simulink model "Over_current_relay"  (R2024a)
settings: Solver=VariableStepAuto  StartTime=0.0  StopTime=10  RelTol=1e-3
libraries: spsACVoltageSourceLib x3, spsGroundLib x3, spsThreePhaseBreakerLib x3, spsVariableRatioTransformerLib x3, spsAsynchronousMachineSIUnitsLib x1, spsCurrentMeasurementLib x1, simulink_extras x1, spsVoltageMeasurementLib x1, sps_lib x1
settings Model: Creator=gshma  LastModifiedBy=gshma

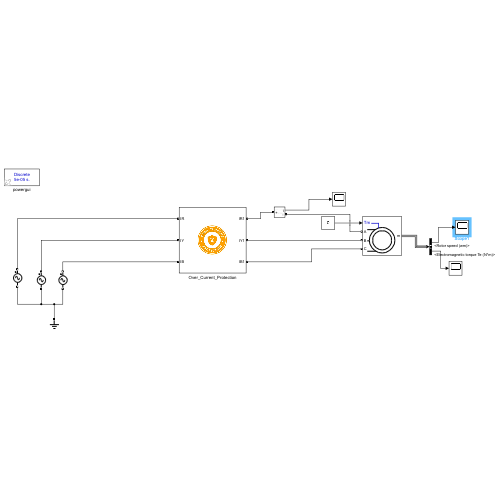
[thumbnail: Simulink's stored preview of the top-level diagram]
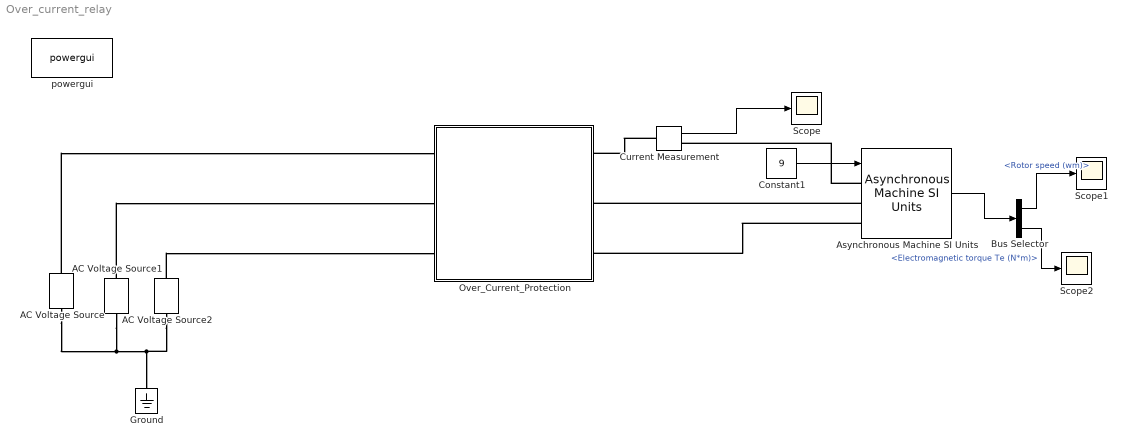
== system Over_current_relay ==
  AC Voltage Source : spsACVoltageSourceLib/AC Voltage Source  Amplitude=400  Phase=0  Frequency=50  SampleTime=0  Measurements=None  BusType=swing  Pref=10e3  Qref=0  Qmin=-inf  Qmax=+inf
  AC Voltage Source1 : spsACVoltageSourceLib/AC Voltage Source  Amplitude=400  Phase=120  Frequency=50  SampleTime=0  Measurements=None  BusType=swing  Pref=10e3  Qref=0  Qmin=-inf  Qmax=+inf
  AC Voltage Source2 : spsACVoltageSourceLib/AC Voltage Source  Amplitude=400  Phase=240  Frequency=50  SampleTime=0  Measurements=None  BusType=swing  Pref=10e3  Qref=0  Qmin=-inf  Qmax=+inf
  Asynchronous Machine SI Units : spsAsynchronousMachineSIUnitsLib/Asynchronous Machine SI Units  RotorType=Squirrel-cage  PresetModel="15:  5.4 HP (4KW)   400 V  50Hz 1430 RPM"  MechanicalLoad=Torque Tm  ShowDetailedParameters=on  ReferenceFrame=Rotor  Units=SI  MeasurementBus=off  NominalParameters=[4000 400 50]  VoltageRatio=1  Stator=[1.405 0.005839]  Rotor=[1.395 0.005839]  Cage1=[0.4155 0.002066]  Cage2=[0.4168 0.0003495]  Lm=0.1722  Mechanical=[0.0131 0.002985 2]  PolePairs=2  InitialConditions=[0 0 0 0 0 0 0 0]  SimulateSaturation=off  Saturation=[14.03593122, 27.81365428, 53.79336849, 72.68890987, 97.98006896, 148.6815601, 215.7428561, 302.9841135, 428.7778367 ; 230, 322, 414, 460, 506, 552, 598, 644, 690]  LoadFlowParameters=1492000  TsPowergui=0  TsBlock=-1  IterativeModel=Trapezoidal non iterative  IterativeDiscreteModel=Trapezoidal non iterative  Pmec=1.492e+006
  Bus Selector : BusSelector  OutputSignals=Mechanical.Rotor speed (wm),Mechanical.Electromagnetic torque Te (N*m)
  Constant1 : Constant  Value=9  SampleTime=0.001
  Current Measurement : spsCurrentMeasurementLib/Current Measurement  PhasorSimulation=off  OutputType=Complex  PSBequivalent=0
  Ground : spsGroundLib/Ground  LConnTagsString=a
  Over_Current_Protection : Subsystem
      mask Display: image('ovv.png', [0,0,0,0,50,50]);
  Scope : Scope
  Scope1 : Scope
  Scope2 : Scope
  powergui : sps_lib/powergui  Priority=1  SimulationMode=Discrete  SampleTime=50e-6  frequency=60  Iterations=50  frequencyindice=50  Pbase=100e6  ErrMax=1e-4  UnitsV=kV  UnitsW=MW  buscounter=0  FunctionMessages=off  echomessages=off  EnableUseOfTLC=off  CurrentSourceSwitches=off  DisableSnubberDevices=off  DisableRonSwitches=off  DisableVfSwitches=off  DisplayEquations=off  AutomaticDiscreteSolvers=off  SolverType=Tustin/Backward Euler (TBE)  Interpol=off  ExternalGateDelay=off  methode=off  Ts=100  x0status=blocks  SPID=on  SwTol=0  HookPort=off  NonlinearTolerance=1e-4  nMaxIteration=100  ContinueOnMaxIteration=off  RestoreLinks=warning  ResistiveCurrentMeasurement=off  Frange=[0:2:500]  Ylog=off  Xlog=on  ShowGrid=off  save=off  variable=ZData  structure=0  ZoomFFT=off  StartTime=0.0  cycles=1  DisplayStyle=1  fundamental=60  FreqAxis=off  MaxFrequency=1000  frequencyindicesteady=1  RmsSteady=1  display=off
  wires:
  Current Measurement/1 -> Scope/1
  Constant1/1 -> Asynchronous Machine SI Units/1
  Asynchronous Machine SI Units/1 -> Bus Selector/1
  Bus Selector/1 -> Scope1/1  "<Rotor speed (wm)>"
  Bus Selector/2 -> Scope2/1  "<Electromagnetic torque Te (N*m)>"
  connections:
  AC Voltage Source/RConn1 -- Over_Current_Protection/LConn1
  AC Voltage Source1/RConn1 -- Over_Current_Protection/LConn2
  AC Voltage Source2/RConn1 -- Over_Current_Protection/LConn3
  Current Measurement/LConn1 -- Over_Current_Protection/RConn1
  Asynchronous Machine SI Units/LConn1 -- Current Measurement/RConn1
  Asynchronous Machine SI Units/LConn2 -- Over_Current_Protection/RConn2
  Asynchronous Machine SI Units/LConn3 -- Over_Current_Protection/RConn3
  AC Voltage Source/LConn1 -- AC Voltage Source1/LConn1 -- AC Voltage Source2/LConn1 -- Ground/LConn1

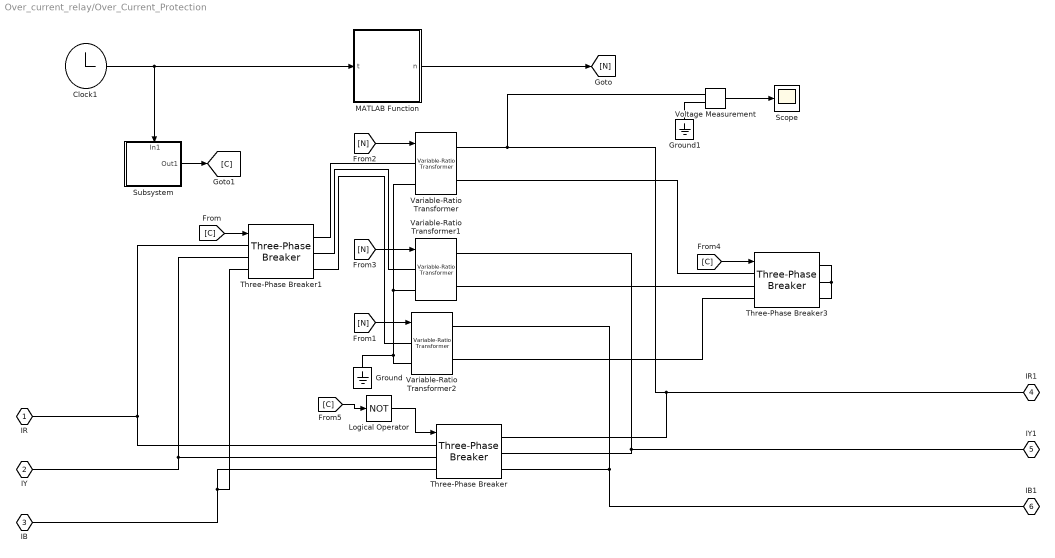
== system Over_current_relay/Over_Current_Protection ==
  Clock1 : Clock
      settings: Decimation=1000
  Ground : spsGroundLib/Ground  LConnTagsString=a
  Ground1 : spsGroundLib/Ground  LConnTagsString=a
  Logical Operator : Logic  Operator=NOT  AllPortsSameDT=off  OutDataTypeStr=boolean
  MATLAB Function : MATLAB Function  TreatAsAtomicUnit=on
  Scope : Scope
  Subsystem : Subsystem
      settings: PortSchema="{\"entries\":[{\"content\":{\"sides\":[{\"content\":{},\"type\":\"ConnectorPlacement.EquallySpacedRectSide\",\"uuid\":\"eeea18b9-380b-488c-afba-283aabc25f85\"},{\"content\":{\"connectorIds\":[\"Out1\"],\"side\":\"RIGHT\"},\"type\":\"ConnectorPlacement.EquallySpacedRectSide\",\"uuid\":\"b5cdad00-14f9-426f-8cac-c80f210bc817\"},{\"content\":{\"connectorIds\":[\"In1\"],\"side\":\"TOP\"},\"type\":\"ConnectorPlacement.EquallySpacedRectSide\",\"uuid\":\"d8660c5f-ab56-4d32-b432-a9ce1bc682f2\"}]},\"type\":\"ConnectorPlacement.EquallySpacedConnector\",\"uuid\":\"80a26fe6-a8a6-4d75-a5f0-c797e7c8950d\"}],\"packageUris\":[\"http://schema.mathworks.com/mf0/Connector/R2020b\"],\"version\":\"1.0\"}"
  Three-Phase Breaker : spsThreePhaseBreakerLib/Three-Phase Breaker  InitialState=open  SwitchA=on  SwitchB=on  SwitchC=on  SwitchTimes="[1/60  5/60]"  External=on  BreakerResistance=0.01  SnubberResistance=1e6  SnubberCapacitance=inf  Measurements=None
  Three-Phase Breaker1 : spsThreePhaseBreakerLib/Three-Phase Breaker  InitialState=closed  SwitchA=on  SwitchB=on  SwitchC=on  SwitchTimes="[1/60  5/60]"  External=on  BreakerResistance=0.01  SnubberResistance=1e6  SnubberCapacitance=inf  Measurements=None
  Three-Phase Breaker3 : spsThreePhaseBreakerLib/Three-Phase Breaker  InitialState=closed  SwitchA=on  SwitchB=on  SwitchC=on  SwitchTimes="[1/60  5/60]"  External=on  BreakerResistance=0.01  SnubberResistance=1e6  SnubberCapacitance=inf  Measurements=None
  Variable-Ratio Transformer : spsVariableRatioTransformerLib/Variable-Ratio Transformer
      settings: LibrarySourceBlock=|
      | sps_lib/Passives/Variable-Ratio
      | Transformer
  Variable-Ratio Transformer1 : spsVariableRatioTransformerLib/Variable-Ratio Transformer
      settings: LibrarySourceBlock=|
      | sps_lib/Passives/Variable-Ratio
      | Transformer
  Variable-Ratio Transformer2 : spsVariableRatioTransformerLib/Variable-Ratio Transformer
      settings: LibrarySourceBlock=|
      | sps_lib/Passives/Variable-Ratio
      | Transformer
  Voltage Measurement : spsVoltageMeasurementLib/Voltage Measurement  PhasorSimulation=off  OutputType=Complex  PSBequivalent=0
  IR : PMIOPort  Tag=simrfV2util1/Connection Port  Side=Left
  IY : PMIOPort  Tag=simrfV2util1/Connection Port  Port=2  Side=Left
  IB : PMIOPort  Tag=simrfV2util1/Connection Port  Port=3  Side=Left
  IR1 : PMIOPort  Tag=simrfV2util1/Connection Port  Port=4  Side=Right
  IY1 : PMIOPort  Tag=simrfV2util1/Connection Port  Port=5  Side=Right
  IB1 : PMIOPort  Tag=simrfV2util1/Connection Port  Port=6  Side=Right
  wires:
  Clock1/1 -> MATLAB Function/1(t), Subsystem/1(In1)
  MATLAB Function/1(n) -> [N]
  [N] -> Variable-Ratio Transformer/1
  [N] -> Variable-Ratio Transformer1/1
  [N] -> Variable-Ratio Transformer2/1
  Subsystem/1(Out1) -> [C]
  [C] -> Three-Phase Breaker1/1
  [C] -> Three-Phase Breaker3/1
  [C] -> Logical Operator/1
  Logical Operator/1 -> Three-Phase Breaker/1
  Voltage Measurement/1 -> Scope/1
  connections:
  Variable-Ratio Transformer/LConn2 -- Ground/LConn1 -- Variable-Ratio Transformer2/LConn2 -- Variable-Ratio Transformer1/LConn2
  Three-Phase Breaker3/LConn1 -- Variable-Ratio Transformer/RConn2
  Three-Phase Breaker3/LConn2 -- Variable-Ratio Transformer1/RConn2
  Three-Phase Breaker3/LConn3 -- Variable-Ratio Transformer2/RConn2
  IR/RConn1 -- Three-Phase Breaker1/LConn1 -- Three-Phase Breaker/LConn1
  IY/RConn1 -- Three-Phase Breaker1/LConn2 -- Three-Phase Breaker/LConn2
  Three-Phase Breaker/LConn3 -- IB/RConn1 -- Three-Phase Breaker1/LConn3
  Three-Phase Breaker3/RConn1 -- Three-Phase Breaker3/RConn3 -- Three-Phase Breaker3/RConn2
  Variable-Ratio Transformer/RConn1 -- Voltage Measurement/LConn1 -- Three-Phase Breaker/RConn1 -- IR1/RConn1
  Variable-Ratio Transformer1/RConn1 -- IY1/RConn1 -- Three-Phase Breaker/RConn2
  Variable-Ratio Transformer2/RConn1 -- Three-Phase Breaker/RConn3 -- IB1/RConn1
  Three-Phase Breaker1/RConn1 -- Variable-Ratio Transformer/LConn1
  Three-Phase Breaker1/RConn2 -- Variable-Ratio Transformer1/LConn1
  Three-Phase Breaker1/RConn3 -- Variable-Ratio Transformer2/LConn1
  Ground1/LConn1 -- Voltage Measurement/LConn2

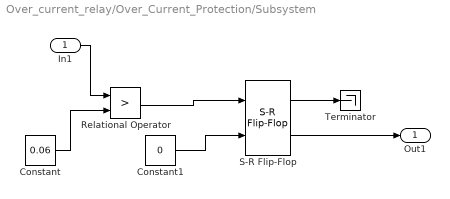
== system Over_current_relay/Over_Current_Protection/Subsystem ==
  In1 : Inport
  Constant : Constant  Value=0.06  SampleTime=0.001
  Constant1 : Constant  Value=0  OutDataTypeStr=boolean  SampleTime=0.0001
  Relational Operator : RelationalOperator  Operator=>  OutDataTypeStr=boolean  RndMeth=Simplest  InputSameDT=off
  S-R Flip-Flop : simulink_extras/Flip Flops/S-R Flip-Flop  initial_condition=0
  Terminator : Terminator
  Out1 : Outport
  wires:
  S-R Flip-Flop/1 -> Terminator/1
  In1/1 -> Relational Operator/1
  Constant/1 -> Relational Operator/2
  Constant1/1 -> S-R Flip-Flop/2
  Relational Operator/1 -> S-R Flip-Flop/1
  S-R Flip-Flop/2 -> Out1/1

== matlab function Over_current_relay/Over_Current_Protection/MATLAB Function ==
  data: t input; n output
function n = fcn(t)
    if t >= 0 && t < 0.03
        n = 0.5;  % Voltage ratio at 50%
    elseif t >=0.03 && t < 0.04
        n = 0.6;  % Voltage ratio at 65%
    else
        n = 0.85;  % Voltage ratio at 80%
    end
end
